simulink model "MN_Renshow_system"  (Simulink 10.2)
settings: Solver=ode45  StartTime=0.0  StopTime=1  RelTol=1e-3  EnableMultiTasking=on
libraries: NeuroModelerLibrary x5
settings Model: Creator=Bakhshiev  LastModifiedBy=Bakhshiev
settings DataIOCC: LimitDataPoints=on
settings OptimizationCC: ExpressionDepthLimit=2147483647  InitFltsAndDblsToZero=on
settings DebuggingCC: SolverPrmCheckMsg=warning  StateNameClashWarn=warning
settings SFSimCC: SimUseLocalCustomCode=on
settings RTWCC: RTWUseLocalCustomCode=on
settings ConfigComp: CovExternalEMLEnable=on

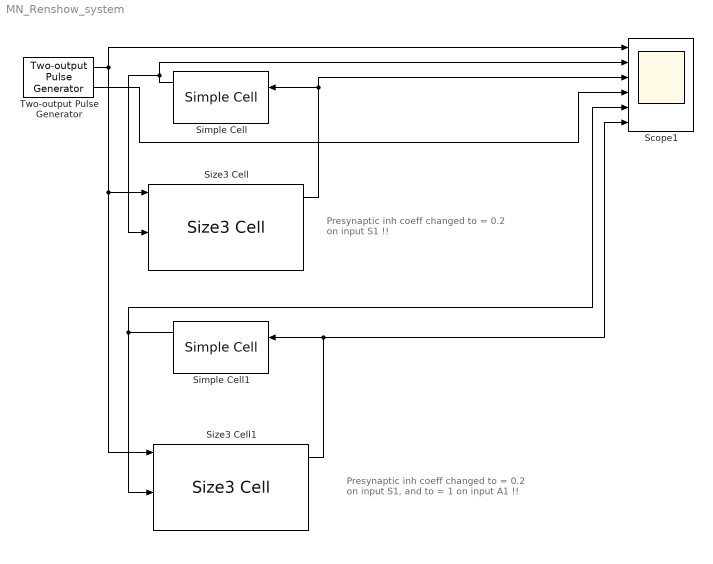
== system MN_Renshow_system ==
  note: Presynaptic inh coeff changed to = 0.2
      | on input S1 !!
  note: Presynaptic inh coeff changed to = 0.2
      | on input S1, and to = 1 on input A1 !!
  Scope1 : Scope  NumInputPorts=6
  Simple Cell : NeuroModelerLibrary/Simple Cells/Simple Cell  SystemSampleTime=-1  VariantActivationTime=update diagram  Latency=0  AutoFrameSizeCalculation=off
  Simple Cell1 : NeuroModelerLibrary/Simple Cells/Simple Cell  SystemSampleTime=-1  VariantActivationTime=update diagram  Latency=0  AutoFrameSizeCalculation=off
  Size3 Cell : NeuroModelerLibrary/Sized Cells/Size3 Cell  SystemSampleTime=-1  VariantActivationTime=update diagram  Latency=0  AutoFrameSizeCalculation=off
      link override Synapse2: ksi=0.2
  Size3 Cell1 : NeuroModelerLibrary/Sized Cells/Size3 Cell  SystemSampleTime=-1  VariantActivationTime=update diagram  Latency=0  AutoFrameSizeCalculation=off
      link override Synapse2: ksi=0.2
      link override Synapse3: ksi=1
  Two-output Pulse Generator : NeuroModelerLibrary/Support/Two-output Pulse Generator  A=1  P1=50  P2=20  PW=1  ST=0.001  OOn1=0.15  OOff1=1  OOn2=0.15  OOff2=1
  wires:
  Size3 Cell/1 -> Scope1/3, Simple Cell/1
  Two-output Pulse Generator/1 -> Scope1/1, Size3 Cell/1, Size3 Cell1/1
  Simple Cell/1 -> Scope1/2, Size3 Cell/5
  Size3 Cell1/1 -> Scope1/6, Simple Cell1/1
  Simple Cell1/1 -> Scope1/5, Size3 Cell1/5
  Two-output Pulse Generator/2 -> Scope1/4
